simulink model "SWC_FRP"  (R2020a)
settings: Solver=FixedStepDiscrete  StartTime=0.0  StopTime=10.0  FixedStep=0.001  RelTol=1e-3
undefined symbols (not defined in the file): CAL_FRP_18VHSVoltRngErrOutCtl_b, CAL_FRP_1V8CPLDVoltRngErrOutCtl_b, CAL_FRP_3V3CPLDVoltRngErrOutCtl_b, CAL_FRP_BMSVoltRngErrOutCtl_b, CAL_FRP_CurrRngErrOutCtl_b, CAL_FRP_CurrSumErrOutCtl_b, CAL_FRP_FaultReactCtl_b, CAL_FRP_iPhasSensVolRngErrOutCtl_b, CAL_FRP_ModeReqRngErrOutCtl_b, CAL_FRP_NSetPRngErrOutCtl_b, CAL_FRP_OffsetRngErrrOutCtl_b, CAL_FRP_RslvExciRngErrOutCtl_b, CAL_FRP_RslvRngErrOutCtl_b, CAL_FRP_RslvSensVolRngErrOutCtl_b, CAL_FRP_RslvSqrtErrOutCtl_b, CAL_FRP_TrqCalcErrOutCtl_b, CAL_FRP_TrqSetPRngErrOutCtl_b, CAL_FRP_UBRVoltRngErrOutCtl_b, CAL_FRP_UintndSpdErrOutCtl_b, CAL_FRP_UintndTrqErrOutCtl_b, CAL_FRP_VoltCmpChkErrOutCtl_b
libraries: hdlsllib x32, simulink x1
settings Model: DataDictionary=SWC_FRP_DataDictionary.sldd  Creator=wangzeda  LastModifiedBy=yangxinqiao
settings DataIOCC: SaveFormat=StructureWithTime
settings OptimizationCC: DefaultParameterBehavior=Inlined  EnhancedBackFolding=on  PassReuseOutputArgsAs=Individual arguments  ZeroExternalMemoryAtStartup=off  ZeroInternalMemoryAtStartup=off  OptimizeBlockOrder=speed  DifferentSizesBufferReuse=on  OptimizationCustomize=off  EfficientTunableParamExpr=on
settings DebuggingCC: ParameterTunabilityLossMsg=error
settings ModelReferenceCC: ModelReferenceNumInstancesAllowed=Single
settings SFSimCC: MATLABDynamicMemAlloc=off
settings RTWCC: SystemTargetFile=ert.tlc  GenCodeOnly=on  TemplateMakefile=ert_default_tmf  CustomSourceCode="#include \"set_get_data.h\""
settings CodeAppCC: ForceParamTrailComments=on  IgnoreCustomStorageClasses=off  OperatorAnnotations=on  SimulinkDataObjDesc=on  SFDataObjDesc=on  InsertBlockDesc=on
settings ERTTargetCC: TargetLangStandard=C99 (ISO)  GenerateASAP2=on  InlinedParameterPlacement=NonHierarchical  ERTCustomFileTemplate=example_file_process.tlc  EnableUserReplacementTypes=on

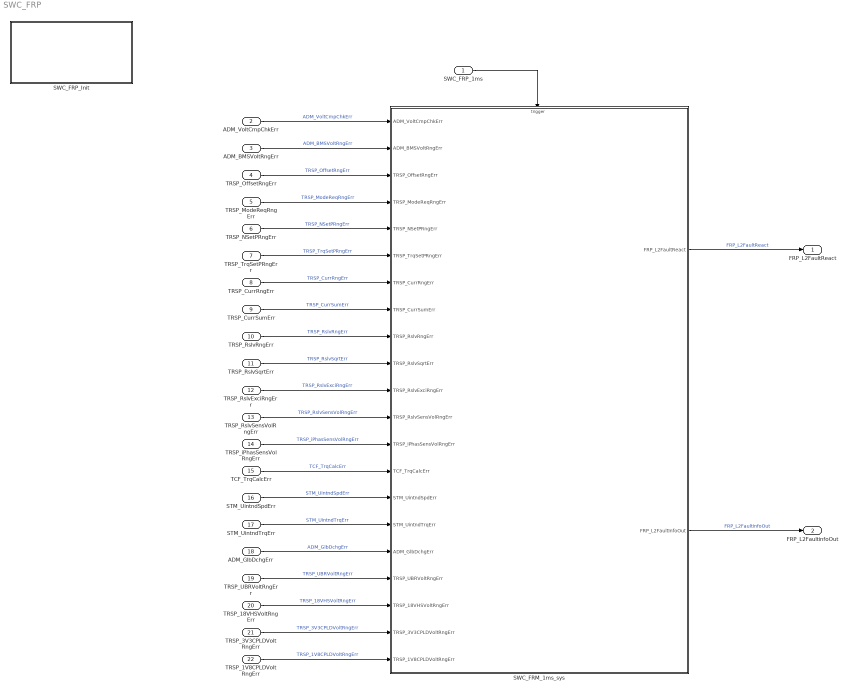
== system SWC_FRP ==
  SWC_FRP_1ms : Inport  SampleTime=0.001  OutputFunctionCall=on
  ADM_VoltCmpChkErr : Inport  Port=2
  ADM_BMSVoltRngErr : Inport  Port=3
  TRSP_OffsetRngErr : Inport  Port=4
  TRSP_ModeReqRngErr : Inport  Port=5
  TRSP_NSetPRngErr : Inport  Port=6
  TRSP_TrqSetPRngErr : Inport  Port=7
  TRSP_CurrRngErr : Inport  Port=8
  TRSP_CurrSumErr : Inport  Port=9
  TRSP_RslvRngErr : Inport  Port=10
  TRSP_RslvSqrtErr : Inport  Port=11
  TRSP_RslvExciRngErr : Inport  Port=12
  TRSP_RslvSensVolRngErr : Inport  Port=13
  TRSP_iPhasSensVolRngErr : Inport  Port=14
  TCF_TrqCalcErr : Inport  Port=15
  STM_UintndSpdErr : Inport  Port=16
  STM_UintndTrqErr : Inport  Port=17
  ADM_GlbDchgErr : Inport  Port=18  OutDataTypeStr=boolean
  TRSP_UBRVoltRngErr : Inport  Port=19  OutDataTypeStr=boolean
  TRSP_18VHSVoltRngErr : Inport  Port=20  OutDataTypeStr=boolean
  TRSP_3V3CPLDVoltRngErr : Inport  Port=21  OutDataTypeStr=boolean
  TRSP_1V8CPLDVoltRngErr : Inport  Port=22  OutDataTypeStr=boolean
  SWC_FRM_1ms_sys : Subsystem
  SWC_FRP_Init : Subsystem
  FRP_L2FaultReact : Outport  OutDataTypeStr=boolean  PortDimensions=1
  FRP_L2FaultinfoOut : Outport  Port=2  OutDataTypeStr=uint32  PortDimensions=1
  wires:
  SWC_FRM_1ms_sys/1(FRP_L2FaultReact) -> FRP_L2FaultReact/1  "FRP_L2FaultReact"
  SWC_FRM_1ms_sys/2(FRP_L2FaultInfoOut) -> FRP_L2FaultinfoOut/1  "FRP_L2FaultinfoOut"
  SWC_FRP_1ms/1 -> SWC_FRM_1ms_sys/Trigger
  TRSP_ModeReqRngErr/1 -> SWC_FRM_1ms_sys/4(TRSP_ModeReqRngErr)  "TRSP_ModeReqRngErr"
  TRSP_NSetPRngErr/1 -> SWC_FRM_1ms_sys/5(TRSP_NSetPRngErr)  "TRSP_NSetPRngErr"
  TRSP_TrqSetPRngErr/1 -> SWC_FRM_1ms_sys/6(TRSP_TrqSetPRngErr)  "TRSP_TrqSetPRngErr"
  TRSP_CurrRngErr/1 -> SWC_FRM_1ms_sys/7(TRSP_CurrRngErr)  "TRSP_CurrRngErr"
  TRSP_CurrSumErr/1 -> SWC_FRM_1ms_sys/8(TRSP_CurrSumErr)  "TRSP_CurrSumErr"
  TRSP_RslvRngErr/1 -> SWC_FRM_1ms_sys/9(TRSP_RslvRngErr)  "TRSP_RslvRngErr"
  TRSP_RslvSqrtErr/1 -> SWC_FRM_1ms_sys/10(TRSP_RslvSqrtErr)  "TRSP_RslvSqrtErr"
  ADM_GlbDchgErr/1 -> SWC_FRM_1ms_sys/17(ADM_GlbDchgErr)  "ADM_GlbDchgErr"
  STM_UintndTrqErr/1 -> SWC_FRM_1ms_sys/16(STM_UintndTrqErr)  "STM_UintndTrqErr"
  STM_UintndSpdErr/1 -> SWC_FRM_1ms_sys/15(STM_UintndSpdErr)  "STM_UintndSpdErr"
  TCF_TrqCalcErr/1 -> SWC_FRM_1ms_sys/14(TCF_TrqCalcErr)  "TCF_TrqCalcErr"
  TRSP_iPhasSensVolRngErr/1 -> SWC_FRM_1ms_sys/13(TRSP_iPhasSensVolRngErr)  "TRSP_iPhasSensVolRngErr"
  TRSP_RslvSensVolRngErr/1 -> SWC_FRM_1ms_sys/12(TRSP_RslvSensVolRngErr)  "TRSP_RslvSensVolRngErr"
  TRSP_RslvExciRngErr/1 -> SWC_FRM_1ms_sys/11(TRSP_RslvExciRngErr)  "TRSP_RslvExciRngErr"
  ADM_BMSVoltRngErr/1 -> SWC_FRM_1ms_sys/2(ADM_BMSVoltRngErr)  "ADM_BMSVoltRngErr"
  TRSP_OffsetRngErr/1 -> SWC_FRM_1ms_sys/3(TRSP_OffsetRngErr)  "TRSP_OffsetRngErr"
  ADM_VoltCmpChkErr/1 -> SWC_FRM_1ms_sys/1(ADM_VoltCmpChkErr)  "ADM_VoltCmpChkErr"
  TRSP_UBRVoltRngErr/1 -> SWC_FRM_1ms_sys/18(TRSP_UBRVoltRngErr)  "TRSP_UBRVoltRngErr"
  TRSP_18VHSVoltRngErr/1 -> SWC_FRM_1ms_sys/19(TRSP_18VHSVoltRngErr)  "TRSP_18VHSVoltRngErr"
  TRSP_3V3CPLDVoltRngErr/1 -> SWC_FRM_1ms_sys/20(TRSP_3V3CPLDVoltRngErr)  "TRSP_3V3CPLDVoltRngErr"
  TRSP_1V8CPLDVoltRngErr/1 -> SWC_FRM_1ms_sys/21(TRSP_1V8CPLDVoltRngErr)  "TRSP_1V8CPLDVoltRngErr"

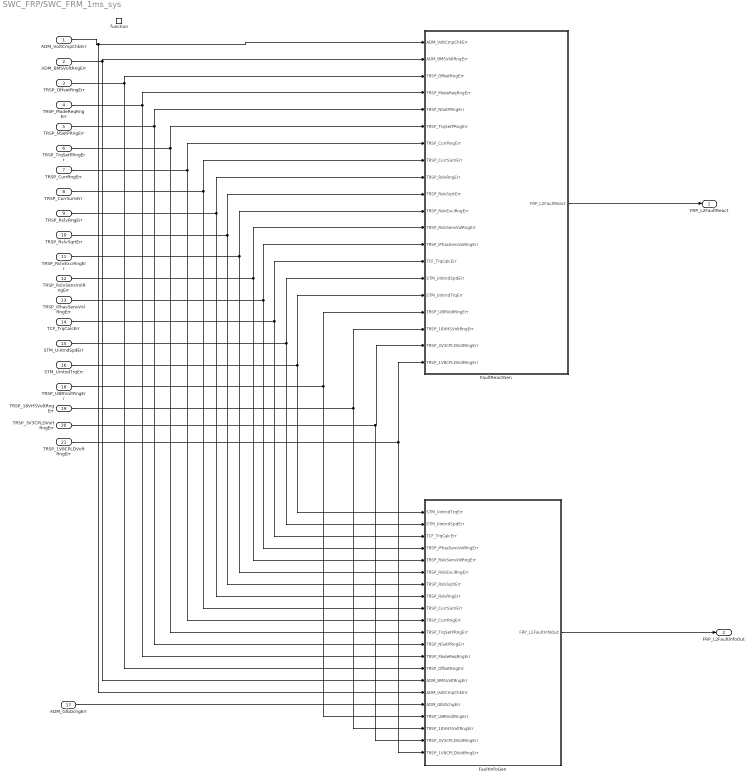
== system SWC_FRP/SWC_FRM_1ms_sys ==
  ADM_VoltCmpChkErr : Inport
  ADM_BMSVoltRngErr : Inport  Port=2
  TRSP_OffsetRngErr : Inport  Port=3
  TRSP_ModeReqRngErr : Inport  Port=4
  TRSP_NSetPRngErr : Inport  Port=5
  TRSP_TrqSetPRngErr : Inport  Port=6
  TRSP_CurrRngErr : Inport  Port=7
  TRSP_CurrSumErr : Inport  Port=8
  TRSP_RslvRngErr : Inport  Port=9
  TRSP_RslvSqrtErr : Inport  Port=10
  TRSP_RslvExciRngErr : Inport  Port=11
  TRSP_RslvSensVolRngErr : Inport  Port=12
  TRSP_iPhasSensVolRngErr : Inport  Port=13
  TCF_TrqCalcErr : Inport  Port=14
  STM_UintndSpdErr : Inport  Port=15
  STM_UintndTrqErr : Inport  Port=16
  ADM_GlbDchgErr : Inport  Port=17
  TRSP_UBRVoltRngErr : Inport  Port=18  OutDataTypeStr=boolean
  TRSP_18VHSVoltRngErr : Inport  Port=19  OutDataTypeStr=boolean
  TRSP_3V3CPLDVoltRngErr : Inport  Port=20  OutDataTypeStr=boolean
  TRSP_1V8CPLDVoltRngErr : Inport  Port=21  OutDataTypeStr=boolean
  function : TriggerPort  TriggerType=function-call  VariantControl=(inherit)  SampleTimeType=periodic  SampleTime=-1
  FaultInfoGen : Subsystem  TreatAsAtomicUnit=on
      settings: RTWSystemCode=Nonreusable function
  FaultReactGen : Subsystem  TreatAsAtomicUnit=on
      settings: RTWSystemCode=Nonreusable function
  FRP_L2FaultReact : Outport
  FRP_L2FaultInfoOut : Outport  Port=2
  wires:
  FaultInfoGen/1(FRP_L2FaultInfoOut) -> FRP_L2FaultInfoOut/1
  FaultReactGen/1(FRP_L2FaultReact) -> FRP_L2FaultReact/1
  ADM_BMSVoltRngErr/1 -> FaultInfoGen/15(ADM_BMSVoltRngErr), FaultReactGen/2(ADM_BMSVoltRngErr)
  TRSP_CurrRngErr/1 -> FaultInfoGen/10(TRSP_CurrRngErr), FaultReactGen/7(TRSP_CurrRngErr)
  TRSP_CurrSumErr/1 -> FaultInfoGen/9(TRSP_CurrSumErr), FaultReactGen/8(TRSP_CurrSumErr)
  TRSP_RslvRngErr/1 -> FaultInfoGen/8(TRSP_RslvRngErr), FaultReactGen/9(TRSP_RslvRngErr)
  TRSP_RslvSqrtErr/1 -> FaultInfoGen/7(TRSP_RslvSqrtErr), FaultReactGen/10(TRSP_RslvSqrtErr)
  TRSP_RslvExciRngErr/1 -> FaultInfoGen/6(TRSP_RslvExciRngErr), FaultReactGen/11(TRSP_RslvExciRngErr)
  TRSP_RslvSensVolRngErr/1 -> FaultInfoGen/5(TRSP_RslvSensVolRngErr), FaultReactGen/12(TRSP_RslvSensVolRngErr)
  TRSP_iPhasSensVolRngErr/1 -> FaultInfoGen/4(TRSP_iPhasSensVolRngErr), FaultReactGen/13(TRSP_iPhasSensVolRngErr)
  TCF_TrqCalcErr/1 -> FaultInfoGen/3(TCF_TrqCalcErr), FaultReactGen/14(TCF_TrqCalcErr)
  TRSP_ModeReqRngErr/1 -> FaultInfoGen/13(TRSP_ModeReqRngErr), FaultReactGen/4(TRSP_ModeReqRngErr)
  TRSP_NSetPRngErr/1 -> FaultInfoGen/12(TRSP_NSetPRngErr), FaultReactGen/5(TRSP_NSetPRngErr)
  TRSP_TrqSetPRngErr/1 -> FaultInfoGen/11(TRSP_TrqSetPRngErr), FaultReactGen/6(TRSP_TrqSetPRngErr)
  STM_UintndSpdErr/1 -> FaultInfoGen/2(STM_UintndSpdErr), FaultReactGen/15(STM_UintndSpdErr)
  STM_UintndTrqErr/1 -> FaultInfoGen/1(STM_UintndTrqErr), FaultReactGen/16(STM_UintndTrqErr)
  ADM_GlbDchgErr/1 -> FaultInfoGen/17(ADM_GlbDchgErr)
  TRSP_OffsetRngErr/1 -> FaultInfoGen/14(TRSP_OffsetRngErr), FaultReactGen/3(TRSP_OffsetRngErr)
  ADM_VoltCmpChkErr/1 -> FaultReactGen/1(ADM_VoltCmpChkErr), FaultInfoGen/16(ADM_VoltCmpChkErr)
  TRSP_UBRVoltRngErr/1 -> FaultInfoGen/18(TRSP_UBRVoltRngErr), FaultReactGen/17(TRSP_UBRVoltRngErr)
  TRSP_18VHSVoltRngErr/1 -> FaultInfoGen/19(TRSP_18VHSVoltRngErr), FaultReactGen/18(TRSP_18VHSVoltRngErr)
  TRSP_3V3CPLDVoltRngErr/1 -> FaultInfoGen/20(TRSP_3V3CPLDVoltRngErr), FaultReactGen/19(TRSP_3V3CPLDVoltRngErr)
  TRSP_1V8CPLDVoltRngErr/1 -> FaultReactGen/20(TRSP_1V8CPLDVoltRngErr), FaultInfoGen/21(TRSP_1V8CPLDVoltRngErr)

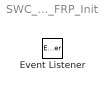
== system SWC_FRP/SWC_FRP_Init ==
  Event Listener : EventListener  EventName=reset

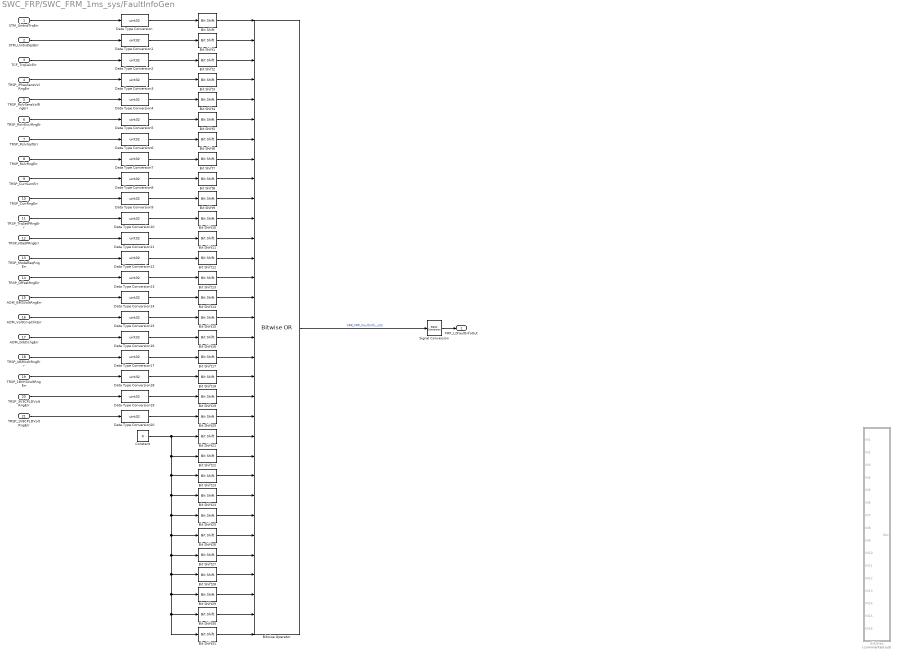
== system SWC_FRP/SWC_FRM_1ms_sys/FaultInfoGen ==
  STM_UintndTrqErr : Inport
  STM_UintndSpdErr : Inport  Port=2
  TCF_TrqCalcErr : Inport  Port=3
  TRSP_iPhasSensVolRngErr : Inport  Port=4
  TRSP_RslvSensVolRngErr : Inport  Port=5
  TRSP_RslvExciRngErr : Inport  Port=6
  TRSP_RslvSqrtErr : Inport  Port=7
  TRSP_RslvRngErr : Inport  Port=8
  TRSP_CurrSumErr : Inport  Port=9
  TRSP_CurrRngErr : Inport  Port=10
  TRSP_TrqSetPRngErr : Inport  Port=11
  TRSP_NSetPRngErr : Inport  Port=12
  TRSP_ModeReqRngErr : Inport  Port=13
  TRSP_OffsetRngErr : Inport  Port=14
  ADM_BMSVoltRngErr : Inport  Port=15
  ADM_VoltCmpChkErr : Inport  Port=16
  ADM_GlbDchgErr : Inport  Port=17
  TRSP_UBRVoltRngErr : Inport  Port=18  OutDataTypeStr=boolean
  TRSP_18VHSVoltRngErr : Inport  Port=19  OutDataTypeStr=boolean
  TRSP_3V3CPLDVoltRngErr : Inport  Port=20  OutDataTypeStr=boolean
  TRSP_1V8CPLDVoltRngErr : Inport  Port=21  OutDataTypeStr=boolean
  Bit Shift : hdlsllib/Logic and Bit Operations/Bit Shift  mode=Shift Left Logical  N=0
  Bit Shift1 : hdlsllib/Logic and Bit Operations/Bit Shift  mode=Shift Left Logical  N=1
  Bit Shift10 : hdlsllib/Logic and Bit Operations/Bit Shift  mode=Shift Left Logical  N=10
  Bit Shift11 : hdlsllib/Logic and Bit Operations/Bit Shift  mode=Shift Left Logical  N=11
  Bit Shift12 : hdlsllib/Logic and Bit Operations/Bit Shift  mode=Shift Left Logical  N=12
  Bit Shift13 : hdlsllib/Logic and Bit Operations/Bit Shift  mode=Shift Left Logical  N=13
  Bit Shift14 : hdlsllib/Logic and Bit Operations/Bit Shift  mode=Shift Left Logical  N=14
  Bit Shift15 : hdlsllib/Logic and Bit Operations/Bit Shift  mode=Shift Left Logical  N=15
  Bit Shift16 : hdlsllib/Logic and Bit Operations/Bit Shift  mode=Shift Left Logical  N=16
  Bit Shift17 : hdlsllib/Logic and Bit Operations/Bit Shift  mode=Shift Left Logical  N=17
  Bit Shift18 : hdlsllib/Logic and Bit Operations/Bit Shift  mode=Shift Left Logical  N=18
  Bit Shift19 : hdlsllib/Logic and Bit Operations/Bit Shift  mode=Shift Left Logical  N=19
  Bit Shift2 : hdlsllib/Logic and Bit Operations/Bit Shift  mode=Shift Left Logical  N=2
  Bit Shift20 : hdlsllib/Logic and Bit Operations/Bit Shift  mode=Shift Left Logical  N=20
  Bit Shift21 : hdlsllib/Logic and Bit Operations/Bit Shift  mode=Shift Left Logical  N=21
  Bit Shift22 : hdlsllib/Logic and Bit Operations/Bit Shift  mode=Shift Left Logical  N=22
  Bit Shift23 : hdlsllib/Logic and Bit Operations/Bit Shift  mode=Shift Left Logical  N=23
  Bit Shift24 : hdlsllib/Logic and Bit Operations/Bit Shift  mode=Shift Left Logical  N=24
  Bit Shift25 : hdlsllib/Logic and Bit Operations/Bit Shift  mode=Shift Left Logical  N=25
  Bit Shift26 : hdlsllib/Logic and Bit Operations/Bit Shift  mode=Shift Left Logical  N=26
  Bit Shift27 : hdlsllib/Logic and Bit Operations/Bit Shift  mode=Shift Left Logical  N=27
  Bit Shift28 : hdlsllib/Logic and Bit Operations/Bit Shift  mode=Shift Left Logical  N=28
  Bit Shift29 : hdlsllib/Logic and Bit Operations/Bit Shift  mode=Shift Left Logical  N=29
  Bit Shift3 : hdlsllib/Logic and Bit Operations/Bit Shift  mode=Shift Left Logical  N=3
  Bit Shift30 : hdlsllib/Logic and Bit Operations/Bit Shift  mode=Shift Left Logical  N=30
  Bit Shift31 : hdlsllib/Logic and Bit Operations/Bit Shift  mode=Shift Left Logical  N=31
  Bit Shift4 : hdlsllib/Logic and Bit Operations/Bit Shift  mode=Shift Left Logical  N=4
  Bit Shift5 : hdlsllib/Logic and Bit Operations/Bit Shift  mode=Shift Left Logical  N=5
  Bit Shift6 : hdlsllib/Logic and Bit Operations/Bit Shift  mode=Shift Left Logical  N=6
  Bit Shift7 : hdlsllib/Logic and Bit Operations/Bit Shift  mode=Shift Left Logical  N=7
  Bit Shift8 : hdlsllib/Logic and Bit Operations/Bit Shift  mode=Shift Left Logical  N=8
  Bit Shift9 : hdlsllib/Logic and Bit Operations/Bit Shift  mode=Shift Left Logical  N=9
  Bit2Hex : Stateflow chart  Commented=on
  Bitwise Operator : simulink/Logic and Bit Operations/Bitwise Operator  logicop=OR  UseBitMask=off  NumInputPorts=32  BitMask=bin2dec('11011001')  BitMaskRealWorld=Stored Integer
  Constant : Constant  Value=0  OutDataTypeStr=uint32
  Data Type Conversion{,1..20} (21 alike) : DataTypeConversion  OutDataTypeStr=uint32
  Signal Conversion : SignalConversion  OverrideOpt=off
  FRP_L2FaultInfoOut : Outport
  wires:
  Bit Shift/1 -> Bitwise Operator/1
  Bit Shift1/1 -> Bitwise Operator/2
  Bit Shift2/1 -> Bitwise Operator/3
  Bit Shift3/1 -> Bitwise Operator/4
  Bit Shift4/1 -> Bitwise Operator/5
  Bit Shift5/1 -> Bitwise Operator/6
  Bit Shift6/1 -> Bitwise Operator/7
  Bit Shift7/1 -> Bitwise Operator/8
  Bit Shift8/1 -> Bitwise Operator/9
  Bit Shift9/1 -> Bitwise Operator/10
  Bit Shift10/1 -> Bitwise Operator/11
  Bit Shift11/1 -> Bitwise Operator/12
  Bit Shift12/1 -> Bitwise Operator/13
  Bit Shift13/1 -> Bitwise Operator/14
  Bit Shift14/1 -> Bitwise Operator/15
  Bit Shift15/1 -> Bitwise Operator/16
  Bit Shift16/1 -> Bitwise Operator/17
  Bit Shift17/1 -> Bitwise Operator/18
  Bit Shift18/1 -> Bitwise Operator/19
  Bit Shift19/1 -> Bitwise Operator/20
  Bit Shift20/1 -> Bitwise Operator/21
  Bit Shift21/1 -> Bitwise Operator/22
  Bit Shift22/1 -> Bitwise Operator/23
  Bit Shift23/1 -> Bitwise Operator/24
  Bit Shift24/1 -> Bitwise Operator/25
  Bit Shift25/1 -> Bitwise Operator/26
  Bit Shift26/1 -> Bitwise Operator/27
  Bit Shift27/1 -> Bitwise Operator/28
  Bit Shift28/1 -> Bitwise Operator/29
  Bit Shift29/1 -> Bitwise Operator/30
  Bit Shift30/1 -> Bitwise Operator/31
  Bit Shift31/1 -> Bitwise Operator/32
  Data Type Conversion/1 -> Bit Shift/1
  Data Type Conversion1/1 -> Bit Shift1/1
  Data Type Conversion2/1 -> Bit Shift2/1
  Data Type Conversion3/1 -> Bit Shift3/1
  Data Type Conversion4/1 -> Bit Shift4/1
  Data Type Conversion5/1 -> Bit Shift5/1
  Data Type Conversion6/1 -> Bit Shift6/1
  Data Type Conversion7/1 -> Bit Shift7/1
  Data Type Conversion8/1 -> Bit Shift8/1
  Data Type Conversion9/1 -> Bit Shift9/1
  Data Type Conversion10/1 -> Bit Shift10/1
  Data Type Conversion11/1 -> Bit Shift11/1
  Data Type Conversion12/1 -> Bit Shift12/1
  Data Type Conversion13/1 -> Bit Shift13/1
  Data Type Conversion14/1 -> Bit Shift14/1
  Data Type Conversion15/1 -> Bit Shift15/1
  Data Type Conversion16/1 -> Bit Shift16/1
  Constant/1 -> Bit Shift22/1, Bit Shift25/1, Bit Shift31/1, Bit Shift30/1, Bit Shift29/1, Bit Shift28/1, Bit Shift27/1, Bit Shift26/1, Bit Shift24/1, Bit Shift23/1, Bit Shift21/1
  ADM_VoltCmpChkErr/1 -> Data Type Conversion15/1
  TRSP_NSetPRngErr/1 -> Data Type Conversion11/1
  TRSP_ModeReqRngErr/1 -> Data Type Conversion12/1
  TRSP_CurrSumErr/1 -> Data Type Conversion8/1
  ADM_BMSVoltRngErr/1 -> Data Type Conversion14/1
  ADM_GlbDchgErr/1 -> Data Type Conversion16/1
  TRSP_TrqSetPRngErr/1 -> Data Type Conversion10/1
  TRSP_OffsetRngErr/1 -> Data Type Conversion13/1
  TRSP_iPhasSensVolRngErr/1 -> Data Type Conversion3/1
  STM_UintndSpdErr/1 -> Data Type Conversion1/1
  TRSP_RslvSensVolRngErr/1 -> Data Type Conversion4/1
  TRSP_RslvExciRngErr/1 -> Data Type Conversion5/1
  TRSP_CurrRngErr/1 -> Data Type Conversion9/1
  TRSP_RslvRngErr/1 -> Data Type Conversion7/1
  TRSP_RslvSqrtErr/1 -> Data Type Conversion6/1
  STM_UintndTrqErr/1 -> Data Type Conversion/1
  TCF_TrqCalcErr/1 -> Data Type Conversion2/1
  Signal Conversion/1 -> FRP_L2FaultInfoOut/1
  Bitwise Operator/1 -> Signal Conversion/1  "VAR_FRP_FaultInfo_u32"
  TRSP_UBRVoltRngErr/1 -> Data Type Conversion17/1
  TRSP_18VHSVoltRngErr/1 -> Data Type Conversion18/1
  TRSP_3V3CPLDVoltRngErr/1 -> Data Type Conversion19/1
  TRSP_1V8CPLDVoltRngErr/1 -> Data Type Conversion20/1
  Data Type Conversion17/1 -> Bit Shift17/1
  Data Type Conversion18/1 -> Bit Shift18/1
  Data Type Conversion19/1 -> Bit Shift19/1
  Data Type Conversion20/1 -> Bit Shift20/1

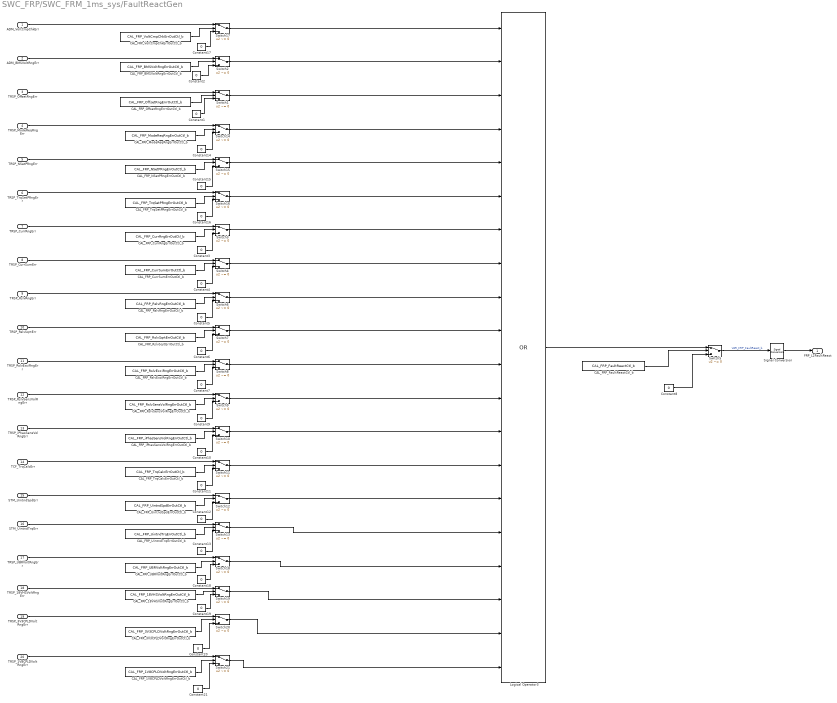
== system SWC_FRP/SWC_FRM_1ms_sys/FaultReactGen ==
  ADM_VoltCmpChkErr : Inport
  ADM_BMSVoltRngErr : Inport  Port=2
  TRSP_OffsetRngErr : Inport  Port=3
  TRSP_ModeReqRngErr : Inport  Port=4
  TRSP_NSetPRngErr : Inport  Port=5
  TRSP_TrqSetPRngErr : Inport  Port=6
  TRSP_CurrRngErr : Inport  Port=7
  TRSP_CurrSumErr : Inport  Port=8
  TRSP_RslvRngErr : Inport  Port=9
  TRSP_RslvSqrtErr : Inport  Port=10
  TRSP_RslvExciRngErr : Inport  Port=11
  TRSP_RslvSensVolRngErr : Inport  Port=12
  TRSP_iPhasSensVolRngErr : Inport  Port=13
  TCF_TrqCalcErr : Inport  Port=14
  STM_UintndSpdErr : Inport  Port=15
  STM_UintndTrqErr : Inport  Port=16
  TRSP_UBRVoltRngErr : Inport  Port=17  OutDataTypeStr=boolean
  TRSP_18VHSVoltRngErr : Inport  Port=18  OutDataTypeStr=boolean
  TRSP_3V3CPLDVoltRngErr : Inport  Port=19  OutDataTypeStr=boolean
  TRSP_1V8CPLDVoltRngErr : Inport  Port=20  OutDataTypeStr=boolean
  CAL_FRP_18VHSVoltRngErrOutCtl_b : Constant  Value=CAL_FRP_18VHSVoltRngErrOutCtl_b  OutDataTypeStr=boolean
  CAL_FRP_1V8CPLDVoltRngErrOutCtl_b : Constant  Value=CAL_FRP_1V8CPLDVoltRngErrOutCtl_b  OutDataTypeStr=boolean
  CAL_FRP_3V3CPLDVoltRngErrOutCtl_b : Constant  Value=CAL_FRP_3V3CPLDVoltRngErrOutCtl_b  OutDataTypeStr=boolean
  CAL_FRP_BMSVoltRngErrOutCtl_b : Constant  Value=CAL_FRP_BMSVoltRngErrOutCtl_b  OutDataTypeStr=boolean
  CAL_FRP_CurrRngErrOutCtl_b : Constant  Value=CAL_FRP_CurrRngErrOutCtl_b  OutDataTypeStr=boolean
  CAL_FRP_CurrSumErrOutCtl_b : Constant  Value=CAL_FRP_CurrSumErrOutCtl_b  OutDataTypeStr=boolean
  CAL_FRP_FaultReactCtl_b : Constant  Value=CAL_FRP_FaultReactCtl_b  OutDataTypeStr=boolean
  CAL_FRP_ModeReqRngErrOutCtl_b : Constant  Value=CAL_FRP_ModeReqRngErrOutCtl_b  OutDataTypeStr=boolean
  CAL_FRP_NSetPRngErrOutCtl_b : Constant  Value=CAL_FRP_NSetPRngErrOutCtl_b  OutDataTypeStr=boolean
  CAL_FRP_OffsetRngErrrOutCtl_b : Constant  Value=CAL_FRP_OffsetRngErrrOutCtl_b  OutDataTypeStr=boolean
  CAL_FRP_RslvExciRngErrOutCtl_b : Constant  Value=CAL_FRP_RslvExciRngErrOutCtl_b  OutDataTypeStr=boolean
  CAL_FRP_RslvRngErrOutCtl_b : Constant  Value=CAL_FRP_RslvRngErrOutCtl_b  OutDataTypeStr=boolean
  CAL_FRP_RslvSensVolRngErrOutCtl_b : Constant  Value=CAL_FRP_RslvSensVolRngErrOutCtl_b  OutDataTypeStr=boolean
  CAL_FRP_RslvSqrtErrOutCtl_b : Constant  Value=CAL_FRP_RslvSqrtErrOutCtl_b  OutDataTypeStr=boolean
  CAL_FRP_TrqCalcErrOutCtl_b : Constant  Value=CAL_FRP_TrqCalcErrOutCtl_b  OutDataTypeStr=boolean
  CAL_FRP_TrqSetPRngErrOutCtl_b : Constant  Value=CAL_FRP_TrqSetPRngErrOutCtl_b  OutDataTypeStr=boolean
  CAL_FRP_UBRVoltRngErrOutCtl_b : Constant  Value=CAL_FRP_UBRVoltRngErrOutCtl_b  OutDataTypeStr=boolean
  CAL_FRP_UintndSpdErrOutCtl_b : Constant  Value=CAL_FRP_UintndSpdErrOutCtl_b  OutDataTypeStr=boolean
  CAL_FRP_UintndTrqErrOutCtl_b : Constant  Value=CAL_FRP_UintndTrqErrOutCtl_b  OutDataTypeStr=boolean
  CAL_FRP_VoltCmpChkErrOutCtl_b : Constant  Value=CAL_FRP_VoltCmpChkErrOutCtl_b  OutDataTypeStr=boolean
  CAL_FRP_iPhasSensVolRngErrOutCtl_b : Constant  Value=CAL_FRP_iPhasSensVolRngErrOutCtl_b  OutDataTypeStr=boolean
  Constant{1..21} (21 alike) : Constant  Value=0  OutDataTypeStr=boolean
  Logical Operator3 : Logic  Operator=OR  Inputs=20  AllPortsSameDT=off  OutDataTypeStr=boolean
  Signal Conversion : SignalConversion  OverrideOpt=off
  Switch{1..21} (21 alike) : Switch  Criteria=u2 ~= 0
  FRP_L2FaultReact : Outport
  wires:
  TRSP_NSetPRngErr/1 -> Switch15/1
  Constant6/1 -> Switch7/3
  Switch16/1 -> Logical Operator3/6
  CAL_FRP_NSetPRngErrOutCtl_b/1 -> Switch15/2
  Constant16/1 -> Switch16/3
  CAL_FRP_ModeReqRngErrOutCtl_b/1 -> Switch14/2
  TRSP_TrqSetPRngErr/1 -> Switch16/1
  ADM_BMSVoltRngErr/1 -> Switch2/1
  Switch15/1 -> Logical Operator3/5
  Switch14/1 -> Logical Operator3/4
  CAL_FRP_RslvSqrtErrOutCtl_b/1 -> Switch7/2
  TRSP_CurrSumErr/1 -> Switch4/1
  TRSP_ModeReqRngErr/1 -> Switch14/1
  TRSP_CurrRngErr/1 -> Switch3/1
  Constant8/1 -> Switch5/3
  Switch13/1 -> Logical Operator3/16
  CAL_FRP_TrqSetPRngErrOutCtl_b/1 -> Switch16/2
  TCF_TrqCalcErr/1 -> Switch11/1
  TRSP_RslvSqrtErr/1 -> Switch7/1
  Constant14/1 -> Switch14/3
  TRSP_RslvSensVolRngErr/1 -> Switch9/1
  Switch10/1 -> Logical Operator3/13
  CAL_FRP_TrqCalcErrOutCtl_b/1 -> Switch11/2
  Constant15/1 -> Switch15/3
  CAL_FRP_UintndTrqErrOutCtl_b/1 -> Switch13/2
  STM_UintndSpdErr/1 -> Switch12/1
  Constant13/1 -> Switch13/3
  CAL_FRP_RslvSensVolRngErrOutCtl_b/1 -> Switch9/2
  Constant2/1 -> Switch2/3
  Logical Operator3/1 -> Switch5/1
  Constant9/1 -> Switch9/3
  Switch2/1 -> Logical Operator3/2
  Switch8/1 -> Logical Operator3/11
  Switch11/1 -> Logical Operator3/14
  Constant5/1 -> Switch6/3
  Constant11/1 -> Switch11/3
  Switch9/1 -> Logical Operator3/12
  Constant4/1 -> Switch4/3
  Switch4/1 -> Logical Operator3/8
  TRSP_RslvExciRngErr/1 -> Switch8/1
  Switch7/1 -> Logical Operator3/10
  Switch6/1 -> Logical Operator3/9
  CAL_FRP_CurrRngErrOutCtl_b/1 -> Switch3/2
  Constant7/1 -> Switch8/3
  Constant10/1 -> Switch10/3
  Switch3/1 -> Logical Operator3/7
  Constant12/1 -> Switch12/3
  CAL_FRP_BMSVoltRngErrOutCtl_b/1 -> Switch2/2
  Switch12/1 -> Logical Operator3/15
  TRSP_iPhasSensVolRngErr/1 -> Switch10/1
  CAL_FRP_CurrSumErrOutCtl_b/1 -> Switch4/2
  TRSP_RslvRngErr/1 -> Switch6/1
  CAL_FRP_RslvExciRngErrOutCtl_b/1 -> Switch8/2
  STM_UintndTrqErr/1 -> Switch13/1
  CAL_FRP_FaultReactCtl_b/1 -> Switch5/2
  Constant3/1 -> Switch3/3
  CAL_FRP_iPhasSensVolRngErrOutCtl_b/1 -> Switch10/2
  CAL_FRP_RslvRngErrOutCtl_b/1 -> Switch6/2
  CAL_FRP_UintndSpdErrOutCtl_b/1 -> Switch12/2
  Switch5/1 -> Signal Conversion/1  "VAR_FRP_FaultReact_b"
  Signal Conversion/1 -> FRP_L2FaultReact/1
  CAL_FRP_OffsetRngErrrOutCtl_b/1 -> Switch1/2
  TRSP_OffsetRngErr/1 -> Switch1/1
  Constant1/1 -> Switch1/3
  Switch1/1 -> Logical Operator3/3
  ADM_VoltCmpChkErr/1 -> Switch17/1
  CAL_FRP_VoltCmpChkErrOutCtl_b/1 -> Switch17/2
  Constant17/1 -> Switch17/3
  Switch17/1 -> Logical Operator3/1
  Constant18/1 -> Switch18/3
  CAL_FRP_UBRVoltRngErrOutCtl_b/1 -> Switch18/2
  TRSP_UBRVoltRngErr/1 -> Switch18/1
  Constant19/1 -> Switch19/3
  CAL_FRP_18VHSVoltRngErrOutCtl_b/1 -> Switch19/2
  CAL_FRP_3V3CPLDVoltRngErrOutCtl_b/1 -> Switch20/2
  Constant20/1 -> Switch20/3
  TRSP_18VHSVoltRngErr/1 -> Switch19/1
  TRSP_3V3CPLDVoltRngErr/1 -> Switch20/1
  CAL_FRP_1V8CPLDVoltRngErrOutCtl_b/1 -> Switch21/2
  Constant21/1 -> Switch21/3
  TRSP_1V8CPLDVoltRngErr/1 -> Switch21/1
  Switch18/1 -> Logical Operator3/17
  Switch19/1 -> Logical Operator3/18
  Switch20/1 -> Logical Operator3/19
  Switch21/1 -> Logical Operator3/20

== stateflow chart SWC_FRP/SWC_FRM_1ms_sys/FaultInfoGen/Bit2Hex ==
  settings: stateMachineType=MEALY_MACHINE
  (default) -> (junction 2)
  (junction 2) -> (junction 4) : {
      | Out=IN16*32768+IN15*16384+IN14*8192+IN13*4096+IN12*2048+IN11*1024+IN10*512+IN9*256+IN8*128+IN7*64+IN6*32+IN5*16+IN4*8+IN3*4+IN2*2+IN1;
      | }
  data: Out output uint16; IN1 input boolean; IN2 input boolean; IN3 input boolean; IN4 input boolean; IN5 input boolean; IN6 input boolean; IN7 input boolean; IN8 input boolean; IN9 input boolean; IN10 input boolean; IN11 input boolean; IN12 input boolean; IN13 input boolean; IN14 input boolean; IN15 input boolean; IN16 input boolean
